simulink model "dcm"  (R2013a)
settings: Solver=ode45  StartTime=0.0  StopTime=3  RelTol=1e-3
values from neighbouring files (symbols this model uses):
  B = 1.24e-4    (= 0.000124)    [dcmsi.m]
  J = 1.1e-4    (= 0.00011)    [dcmsi.m]
  ke = 0.038    [dcmsi.m]
  kt = 0.038    [dcmsi.m]
  kTwl = -5e-4    (= -0.0005)    [dcmsi.m]
  La = 6.67e-4    (= 0.000667)    [dcmsi.m]
  Ra = 1.6    [dcmsi.m]
  V = 24    [dcmsi.m]
settings Model: Creator=dello  LastModifiedBy=dello
settings SolverCC: SolverResetMethod=Robust
settings DataIOCC: SignalLoggingSaveFormat=ModelDataLogs  SignalLoggingName=results
settings OptimizationCC: BlockReduction=off
settings DebuggingCC: UnconnectedInputMsg=none  UnconnectedOutputMsg=none  UnconnectedLineMsg=none

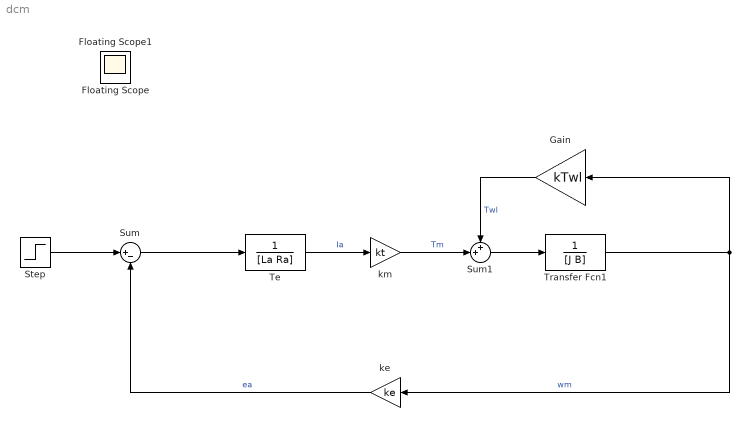
== system dcm ==
  Gain : Gain  Gain=kTwl
  Step : Step  After=V  SampleTime=0
  Sum : Sum  Inputs=|+-
  Sum1 : Sum  Inputs=++|
  Te : TransferFcn  Denominator=[La Ra]
  Transfer Fcn1 : TransferFcn  Denominator=[J B]
  ke : Gain  Gain=ke
  km : Gain  Gain=kt
  Floating Scope : Scope  NumInputPorts=8
      settings: Floating=on  TimeRange=0.03333333333333333  YMin=-5~-5~-5~-5~-5~-5~-5~-5  YMax=5~5~5~5~5~5~5~5  SaveName=diodes
  Floating Scope1 : Scope
      settings: Floating=on  TimeRange=0.03333333333333333  SaveName=simdata
  wires:
  Sum/1 -> Te/1
  Te/1 -> km/1  "Ia"
  km/1 -> Sum1/2  "Tm"
  Sum1/1 -> Transfer Fcn1/1
  Transfer Fcn1/1 -> ke/1, Gain/1  "wm"
  ke/1 -> Sum/2  "ea"
  Step/1 -> Sum/1
  Gain/1 -> Sum1/1  "Twl"
